simulink library "IGStatus"  (R2015a)
settings: Solver=ode45  StartTime=0.0  StopTime=10.0  RelTol=1e-3
values from neighbouring files (symbols this model uses):
  IGVoltage_OFF = uint8(204)    [params.m]
  IGVoltage_ON = uint8(307)    [params.m]
settings Model: Creator=mbd_user  LastModifiedBy=mbd_user

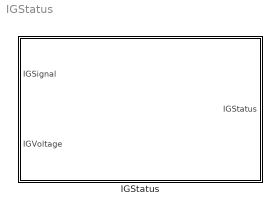
== system IGStatus ==
  IGStatus : Subsystem  TreatAsAtomicUnit=on

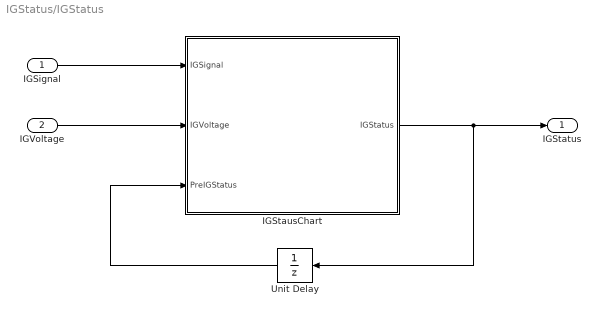
== system IGStatus/IGStatus ==
  IGSignal : Inport
  IGVoltage : Inport  Port=2
  IGStausChart : Stateflow chart  TreatAsAtomicUnit=on
  Unit Delay : UnitDelay  InitialCondition=OFF  SampleTime=-1
      settings: AttributesFormatString=Initial=%<InitialCondition>
  IGStatus : Outport
  wires:
  IGSignal/1 -> IGStausChart/1(IGSignal)
  IGVoltage/1 -> IGStausChart/2(IGVoltage)
  IGStausChart/1(IGStatus) -> Unit Delay/1, IGStatus/1
  Unit Delay/1 -> IGStausChart/3(PreIGStatus)

== stateflow chart IGStatus/IGStausChart ==
  (default) -> (junction 11) : {IGStatus = PreIGStatus}
  (junction 11) -> (junction 12) [order 1] : [IGSignal == ON && IGVoltage >= IGVoltage_ON]
  (junction 11) -> (junction 16) [order 2]
  (junction 12) -> (junction 23) : {IGStatus = ON;}
  (junction 16) -> (junction 19) [order 1] : [IGSignal == OFF && IGVoltage < IGVoltage_OFF]
  (junction 16) -> (junction 21) [order 2]
  (junction 19) -> (junction 22) : {IGStatus = OFF;}
  (junction 22) -> (junction 21)
  (junction 23) -> (junction 22)
  (junction 21) -> (junction 29)
  data: IGSignal input; IGVoltage input; IGStatus output uint8; PreIGStatus input; ON parameter; OFF parameter; IGVoltage_ON parameter; IGVoltage_OFF parameter
